simulink model "bike_model"  (R2018a)
settings: Solver=FixedStepAuto  StartTime=0.0  StopTime=10  FixedStep=Ts_IMU  RelTol=1e-3
values from neighbouring files (symbols this model uses):
  A_full = zeros(length(velocity_lqr),3,3)    [bike_init.m]
  A_full_dis = zeros(length(velocity_lqr),3,3)    [bike_init.m]
  amp_dist_roll_rate = 1    [bike_init.m]
  b = 1.095    [bike_init.m]    (also in bike_init_Merged_v1.m = bike3D190215())
  B_full = zeros(length(velocity_lqr),3)    [bike_init.m]
  B_full_dis = zeros(length(velocity_lqr),3)    [bike_init.m]
  C = eye(3)    [bike_init.m]    (also in bike_init_Merged_v1.m)
  complementary = 0.995    [bike_init.m]    (also in bike_init_Merged_v1.m = 0.985)
  cumulative_dist_along_path = [0;cumsum(dist_from_vertex_to_vertex,1)]    [bike_init.m]    (also in bike_init_Merged_v1.m)
  Dead_Band = [0.055,-0.005,0.005]    [bike_init.m]    (also in bike_init_Merged_v1.m = [0.055,-0.055,0.005])
  delay = 0.045    [bike_init.m]    (also in bike_init_Merged_v1.m)
  discrete = 1    [bike_init.m]
  dist_freq = 100    [bike_init.m]
  g = 9.81    [bike_init.m]    (also in bike_init_Merged_v1.m)
  IMU_height = 0.9    [bike_init.m]
  initial_x = x_ini_diff    (= 0)    [bike_init.m]    (also in bike_init_Merged_v1.m)
  initial_y = y_ini_diff    (= 0)    [bike_init.m]    (also in bike_init_Merged_v1.m)
  input_velocity = 2    [bike_init.m]    (also in bike_init_Merged_v1.m = 2.5)
  K_full = zeros(length(velocity_lqr),3)    [bike_init.m]
  K_full_dis = zeros(length(velocity_lqr),3)    [bike_init.m]    (also in bike_init_Merged_v1.m)
  L_full = zeros(length(velocity_lqr),3,3)    [bike_init.m]
  L_full_dis = zeros(length(velocity_lqr),3,3)    [bike_init.m]
  max_handlebar = 40*(pi/180)    (= 0.698131700798)    [bike_init.m]    (also in bike_init_Merged_v1.m)
  max_steering_motor_acc = inf    [bike_init.m]    (also in bike_init_Merged_v1.m)
  max_steering_motor_speed = 7.5    [bike_init.m]    (also in bike_init_Merged_v1.m)
  min_handlebar = -max_handlebar    (= -0.698131700798)    [bike_init.m]    (also in bike_init_Merged_v1.m)
  min_steering_motor_acc = -inf    [bike_init.m]    (also in bike_init_Merged_v1.m)
  min_steering_motor_speed = -7.5    [bike_init.m]    (also in bike_init_Merged_v1.m)
  noise_acc = 0.006*(pi/180)    (= 0.00010471975512)    [bike_init.m]    (also in bike_init_Merged_v1.m)
  noise_encoder = 1e-7    (= 1e-07)    [bike_init.m]    (also in bike_init_Merged_v1.m)
  noise_gyro = 0.001929307*(pi/180)    (= 3.36727594318e-05)    [bike_init.m]    (also in bike_init_Merged_v1.m)
  noise_hall = 0    [bike_init.m]    (also in bike_init_Merged_v1.m)
  parameters = [g h b a]    [bike_init.m]
  path_x = time_array    [bike_init.m]    (also in bike_init_Merged_v1.m)
  path_y = sqrt(path_x * 0.8) .* sin(0.1*path_x)    [bike_init.m]    (also in bike_init_Merged_v1.m)
  roll_rate_coef = 0.8    [bike_init.m]    (also in bike_init_Merged_v1.m = 0.9)
  Ts = 0.04    [bike_init.m]    (also in bike_init_Merged_v1.m)
  Ts_IMU = 0.01    [bike_init.m]    (also in bike_init_Merged_v1.m = 0.04)
  velocity_lqr = linspace(0.001,10,100)    [bike_init.m]    (also in bike_init_Merged_v1.m = [velocity_lqr-0.1 velocity_lqr velocity_lqr+0.1])
undefined symbols (not defined in the file or in its folder): curvature
libraries: simulink x14, dspsigops x2, dspsigattribs x1
(part 3 of 3)

== system bike_model/State Estimator/B (continuous) ==
  Velocity : Inport
  1-D Lookup Table10 : Lookup_n-D  NumberOfTableDimensions=1  BreakpointsForDimension1=velocity_lqr  BreakpointsForDimension2=velocity_lqr  BreakpointsForDimension3=velocity_lqr  BreakpointsForDimension4=velocity_lqr  Table=B_full(:,2)  InternalRulePriority=Speed  RndMeth=Simplest  InputSameDT=on
  1-D Lookup Table11 : Lookup_n-D  NumberOfTableDimensions=1  BreakpointsForDimension1=velocity_lqr  BreakpointsForDimension2=velocity_lqr  BreakpointsForDimension3=velocity_lqr  BreakpointsForDimension4=velocity_lqr  Table=B_full(:,3)  InternalRulePriority=Speed  RndMeth=Simplest  InputSameDT=on
  1-D Lookup Table3 : Lookup_n-D  NumberOfTableDimensions=1  BreakpointsForDimension1=velocity_lqr  BreakpointsForDimension2=velocity_lqr  BreakpointsForDimension3=velocity_lqr  BreakpointsForDimension4=velocity_lqr  Table=B_full(:,1)  InternalRulePriority=Speed  RndMeth=Simplest  InputSameDT=on
  Display1 : Display
  Matrix Concatenate3 : Concatenate  NumInputs=3  Mode=Multidimensional array
  B : Outport
  wires:
  1-D Lookup Table11/1 -> Matrix Concatenate3/3  "B3"
  Velocity/1 -> 1-D Lookup Table3/1, 1-D Lookup Table11/1, 1-D Lookup Table10/1
  1-D Lookup Table3/1 -> Matrix Concatenate3/1  "B1"
  1-D Lookup Table10/1 -> Matrix Concatenate3/2  "B2"
  Matrix Concatenate3/1 -> Display1/1, B/1

== system bike_model/IMU with complementary filter/Accelerometer/Centripetal Acceleration Compensator ==
  Steering Angle : Inport
  Velocity : Inport  Port=2
  Divide : Product  Inputs=*/
  Multiply : Product
  Square : Math  Operator=square  SaturateOnIntegerOverflow=on
  Tan : Trigonometry  Operator=tan
  b : Constant  Value=b
  Estimated Centripetal Acceleration : Outport
  wires:
  Velocity/1 -> Square/1
  Square/1 -> Divide/1
  b/1 -> Divide/2
  Steering Angle/1 -> Tan/1
  Divide/1 -> Multiply/1
  Tan/1 -> Multiply/2
  Multiply/1 -> Estimated Centripetal Acceleration/1

== system bike_model/IMU with complementary filter/Accelerometer/Lateral Acceleration Compensator ==
  Roll Rate : Inport
  Constant4 : Constant  Value=IMU_height
  Low Pass Filter : Subsystem
  Multiply1 : Product
  Numerical Derivative : Subsystem
  Estimated Lateral Accelerattion due to Roll : Outport
  wires:
  Numerical Derivative/1(Roll Acceleration) -> Multiply1/2  "angular acceleration"
  Roll Rate/1 -> Low Pass Filter/1(Roll Rate)
  Constant4/1 -> Multiply1/1
  Multiply1/1 -> Estimated Lateral Accelerattion due to Roll/1  "lateral acceleration"
  Low Pass Filter/1(Filtered Roll Rate) -> Numerical Derivative/1(Roll Rate)

== system bike_model/IMU with complementary filter wit no centripetal compensation/Accelerometer/Centripetal Acceleration Compensator ==
  Steering Angle : Inport
  Velocity : Inport  Port=2
  Divide : Product  Inputs=*/
  Multiply : Product
  Square : Math  Operator=square  SaturateOnIntegerOverflow=on
  Tan : Trigonometry  Operator=tan
  b : Constant  Value=b
  Estimated Centripetal Acceleration : Outport
  wires:
  Velocity/1 -> Square/1
  Square/1 -> Divide/1
  b/1 -> Divide/2
  Steering Angle/1 -> Tan/1
  Divide/1 -> Multiply/1
  Tan/1 -> Multiply/2
  Multiply/1 -> Estimated Centripetal Acceleration/1

== system bike_model/IMU with complementary filter wit no centripetal compensation/Accelerometer/Lateral Acceleration Compensator ==
  Roll Rate : Inport
  Constant4 : Constant  Value=IMU_height
  Low Pass Filter : Subsystem
  Multiply1 : Product
  Numerical Derivative : Subsystem
  Scope : Scope  NumInputPorts=2
  Scope1 : Scope
  Estimated Lateral Accelerattion due to Roll : Outport
  wires:
  Numerical Derivative/1(Roll Acceleration) -> Scope1/1, Multiply1/2  "angular acceleration"
  Roll Rate/1 -> Scope/1, Low Pass Filter/1(Roll Rate)
  Constant4/1 -> Multiply1/1
  Multiply1/1 -> Estimated Lateral Accelerattion due to Roll/1  "lateral acceleration"
  Low Pass Filter/1(Filtered Roll Rate) -> Scope/2, Numerical Derivative/1(Roll Rate)

== system bike_model/IMU with complementary filter wit no compensation/Accelerometer/Centripetal Acceleration Compensator ==
  Steering Angle : Inport
  Velocity : Inport  Port=2
  Divide : Product  Inputs=*/
  Multiply : Product
  Square : Math  Operator=square  SaturateOnIntegerOverflow=on
  Tan : Trigonometry  Operator=tan
  b : Constant  Value=b
  Estimated Centripetal Acceleration : Outport
  wires:
  Velocity/1 -> Square/1
  Square/1 -> Divide/1
  b/1 -> Divide/2
  Steering Angle/1 -> Tan/1
  Divide/1 -> Multiply/1
  Tan/1 -> Multiply/2
  Multiply/1 -> Estimated Centripetal Acceleration/1

== system bike_model/IMU with complementary filter wit no compensation/Accelerometer/Lateral Acceleration Compensator ==
  Roll Rate : Inport
  Constant4 : Constant  Value=IMU_height
  Low Pass Filter : Subsystem
  Multiply1 : Product
  Numerical Derivative : Subsystem
  Estimated Lateral Accelerattion due to Roll : Outport
  wires:
  Numerical Derivative/1(Roll Acceleration) -> Multiply1/2  "angular acceleration"
  Roll Rate/1 -> Low Pass Filter/1(Roll Rate)
  Constant4/1 -> Multiply1/1
  Multiply1/1 -> Estimated Lateral Accelerattion due to Roll/1  "lateral acceleration"
  Low Pass Filter/1(Filtered Roll Rate) -> Numerical Derivative/1(Roll Rate)

== system bike_model/IMU with complementary filter wit no roll compensation/Accelerometer/Centripetal Acceleration Compensator ==
  Steering Angle : Inport
  Velocity : Inport  Port=2
  Divide : Product  Inputs=*/
  Multiply : Product
  Square : Math  Operator=square  SaturateOnIntegerOverflow=on
  Tan : Trigonometry  Operator=tan
  b : Constant  Value=b
  Estimated Centripetal Acceleration : Outport
  wires:
  Velocity/1 -> Square/1
  Square/1 -> Divide/1
  b/1 -> Divide/2
  Steering Angle/1 -> Tan/1
  Divide/1 -> Multiply/1
  Tan/1 -> Multiply/2
  Multiply/1 -> Estimated Centripetal Acceleration/1

== system bike_model/IMU with complementary filter wit no roll compensation/Accelerometer/Lateral Acceleration Compensator ==
  Roll Rate : Inport
  Constant4 : Constant  Value=IMU_height
  Low Pass Filter : Subsystem
  Multiply1 : Product
  Numerical Derivative : Subsystem
  Estimated Lateral Accelerattion due to Roll : Outport
  wires:
  Numerical Derivative/1(Roll Acceleration) -> Multiply1/2  "angular acceleration"
  Roll Rate/1 -> Low Pass Filter/1(Roll Rate)
  Constant4/1 -> Multiply1/1
  Multiply1/1 -> Estimated Lateral Accelerattion due to Roll/1  "lateral acceleration"
  Low Pass Filter/1(Filtered Roll Rate) -> Numerical Derivative/1(Roll Rate)

== system bike_model/IMU with complementary filter/Accelerometer/Lateral Acceleration Compensator/Low Pass Filter ==
  Roll Rate : Inport
  Delay18 : Delay  DelayLength=1
  Gain4 : Gain  Gain=roll_rate_coef
  Gain6 : Gain  Gain=1-roll_rate_coef
  Scope7 : Scope  NumInputPorts=2
  Sum4 : Sum  Inputs=|++
  Filtered Roll Rate : Outport
  wires:
  Gain6/1 -> Sum4/1
  Gain4/1 -> Sum4/2
  Sum4/1 -> Filtered Roll Rate/1, Delay18/1, Scope7/2  "Filtered Roll Rate"
  Delay18/1 -> Gain4/1
  Roll Rate/1 -> Scope7/1, Gain6/1  "Measured Roll Rate"

== system bike_model/IMU with complementary filter/Accelerometer/Lateral Acceleration Compensator/Numerical Derivative ==
  Roll Rate : Inport
  Delay18 : Delay  DelayLength=1
  Gain3 : Gain  Gain=1/Ts_IMU
  Sum3 : Sum  Inputs=|+-
  Roll Acceleration : Outport
  wires:
  Sum3/1 -> Gain3/1
  Delay18/1 -> Sum3/2
  Roll Rate/1 -> Sum3/1, Delay18/1
  Gain3/1 -> Roll Acceleration/1

== system bike_model/IMU with complementary filter wit no centripetal compensation/Accelerometer/Lateral Acceleration Compensator/Low Pass Filter ==
  Roll Rate : Inport
  Delay18 : Delay  DelayLength=1
  Gain4 : Gain  Gain=roll_rate_coef
  Gain6 : Gain  Gain=1-roll_rate_coef
  Scope7 : Scope  NumInputPorts=2
  Sum4 : Sum  Inputs=|++
  Filtered Roll Rate : Outport
  wires:
  Gain6/1 -> Sum4/1
  Gain4/1 -> Sum4/2
  Sum4/1 -> Filtered Roll Rate/1, Delay18/1, Scope7/2  "Filtered Roll Rate"
  Delay18/1 -> Gain4/1
  Roll Rate/1 -> Scope7/1, Gain6/1  "Measured Roll Rate"

== system bike_model/IMU with complementary filter wit no centripetal compensation/Accelerometer/Lateral Acceleration Compensator/Numerical Derivative ==
  Roll Rate : Inport
  Delay18 : Delay  DelayLength=1
  Gain3 : Gain  Gain=1/Ts_IMU
  Sum3 : Sum  Inputs=|+-
  Roll Acceleration : Outport
  wires:
  Sum3/1 -> Gain3/1
  Delay18/1 -> Sum3/2
  Roll Rate/1 -> Sum3/1, Delay18/1
  Gain3/1 -> Roll Acceleration/1

== system bike_model/IMU with complementary filter wit no compensation/Accelerometer/Lateral Acceleration Compensator/Low Pass Filter ==
  Roll Rate : Inport
  Delay18 : Delay  DelayLength=1
  Gain4 : Gain  Gain=roll_rate_coef
  Gain6 : Gain  Gain=1-roll_rate_coef
  Scope7 : Scope  NumInputPorts=2
  Sum4 : Sum  Inputs=|++
  Filtered Roll Rate : Outport
  wires:
  Gain6/1 -> Sum4/1
  Gain4/1 -> Sum4/2
  Sum4/1 -> Filtered Roll Rate/1, Delay18/1, Scope7/2  "Filtered Roll Rate"
  Delay18/1 -> Gain4/1
  Roll Rate/1 -> Scope7/1, Gain6/1  "Measured Roll Rate"

== system bike_model/IMU with complementary filter wit no compensation/Accelerometer/Lateral Acceleration Compensator/Numerical Derivative ==
  Roll Rate : Inport
  Delay18 : Delay  DelayLength=1
  Gain3 : Gain  Gain=1/Ts_IMU
  Sum3 : Sum  Inputs=|+-
  Roll Acceleration : Outport
  wires:
  Sum3/1 -> Gain3/1
  Delay18/1 -> Sum3/2
  Roll Rate/1 -> Sum3/1, Delay18/1
  Gain3/1 -> Roll Acceleration/1

== system bike_model/IMU with complementary filter wit no roll compensation/Accelerometer/Lateral Acceleration Compensator/Low Pass Filter ==
  Roll Rate : Inport
  Delay18 : Delay  DelayLength=1
  Gain4 : Gain  Gain=roll_rate_coef
  Gain6 : Gain  Gain=1-roll_rate_coef
  Scope7 : Scope  NumInputPorts=2
  Sum4 : Sum  Inputs=|++
  Filtered Roll Rate : Outport
  wires:
  Gain6/1 -> Sum4/1
  Gain4/1 -> Sum4/2
  Sum4/1 -> Filtered Roll Rate/1, Delay18/1, Scope7/2  "Filtered Roll Rate"
  Delay18/1 -> Gain4/1
  Roll Rate/1 -> Scope7/1, Gain6/1  "Measured Roll Rate"

== system bike_model/IMU with complementary filter wit no roll compensation/Accelerometer/Lateral Acceleration Compensator/Numerical Derivative ==
  Roll Rate : Inport
  Delay18 : Delay  DelayLength=1
  Gain3 : Gain  Gain=1/Ts_IMU
  Sum3 : Sum  Inputs=|+-
  Roll Acceleration : Outport
  wires:
  Sum3/1 -> Gain3/1
  Delay18/1 -> Sum3/2
  Roll Rate/1 -> Sum3/1, Delay18/1
  Gain3/1 -> Roll Acceleration/1

== matlab function bike_model/Reference States/Reference Roll Angle Calculator ==
  data: parameters input; velocity input; delta_ref input; phi_ref output
function phi_ref = fcn(parameters, velocity, delta_ref)
g = parameters(1);
b = parameters(3);
v = velocity;

phi_ref = atan(v^2 / (g * b) * delta_ref); % tan(theta_ref));

== matlab function bike_model/Global Angles and Coordinates/Measured Bike Angles to Global Angles/MATLAB Function ==
  data: v input; parameters input; delta input; psi_d output; beta output
function [psi_d, beta]  = fcn(v, parameters, delta)

b = parameters(3);
a = parameters(4);

beta = atan((a / (b)) * tan(delta));
psi_d = (v / a) * sin(beta);

== matlab function bike_model/Reference Position and Direction in Global CS with variable Look Ahead/Look-Ahead Coefficient Modifier (Slow Turn-Off)  ==
  data: look_ahead input; look_ahead_modified output; feedback input; time input; time_delayed input
function look_ahead_modified = fcn(look_ahead, feedback, time, time_delayed)

step=time-time_delayed;

kill_time=3;

delta=(feedback*step)/kill_time;

if look_ahead-feedback<-0.0001
    look_ahead_modified=feedback-delta;
else
    look_ahead_modified = look_ahead;
end
    

end

== matlab function bike_model/Global Angles and Coordinates/Measured Global Angles to Global Coordinates/MATLAB Function1 ==
  data: v input; psi input; Xdot output; beta input; Ydot output
function [Xdot, Ydot]  = fcn(v, psi, beta)

Xdot = v * cos(psi + beta);
Ydot = v * sin(psi + beta);

== matlab function bike_model/Reference Position and Direction in Global CS with variable Look Ahead/Look-Ahead Coefficient Selector ==
  data: curv_next input; look_ahead output; curv input
function look_ahead = fcn(curv_next, curv)


if curv>-0.01 && curv<0.01
    curv=0;
end

if curv_next>-0.01 && curv_next<0.01
    curv_next=0;
end



if curv>=0
    if curv-curv_next>0
        look_ahead=0;
    else
        look_ahead=curv_next-curv;
    end
else
    if curv-curv_next<0
        look_ahead=0;
    else
        look_ahead=curv-curv_next;
    end
end



end

== matlab function bike_model/Global Angles and Coordinates/True Bike Angles to Global Angles2/MATLAB Function ==
  data: v input; parameters input; delta input; psi_d output; beta output
function [psi_d, beta]  = fcn(v, parameters, delta)

b = parameters(3);
a = parameters(4);

beta = atan((a / (b)) * tan(delta));
psi_d = (v / a) * sin(beta);

== matlab function bike_model/Global Angles and Coordinates/True Global Angles to Global Coordinates/MATLAB Function1 ==
  data: v input; psi input; Xdot output; beta input; Ydot output
function [Xdot, Ydot]  = fcn(v, psi, beta)

Xdot = v * cos(psi + beta);
Ydot = v * sin(psi + beta);
